simulink model "td1jacobian"  (R2024a)
settings: Solver=FixedStepAuto  StartTime=0.0  StopTime=10.0  FixedStep=0.01  RelTol=1e-3
settings Model: Creator=tr_nguye  LastModifiedBy=tr_nguye

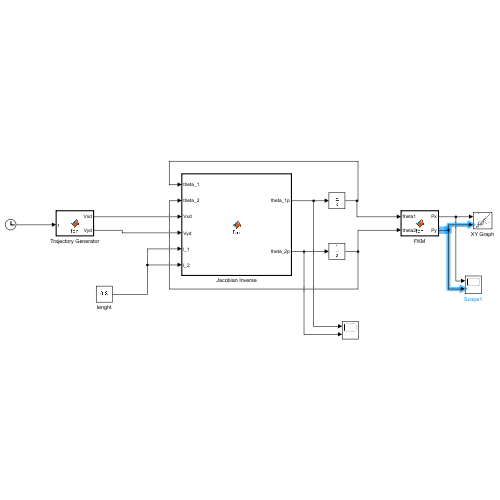
[thumbnail: Simulink's stored preview of the top-level diagram]
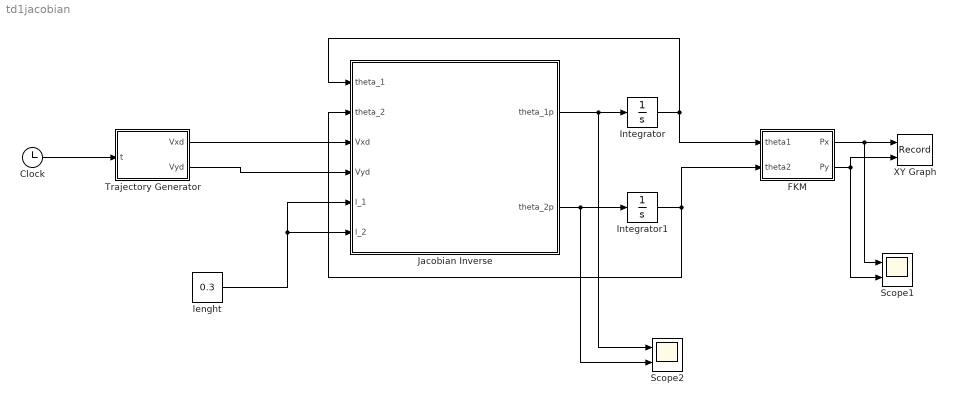
== system td1jacobian ==
  Clock : Clock
      settings: Decimation=1000
  FKM : MATLAB Function  TreatAsAtomicUnit=on
  Integrator : Integrator  InitialCondition=-1.2683
  Integrator1 : Integrator  InitialCondition=0.4759
  Jacobian Inverse : MATLAB Function  TreatAsAtomicUnit=on
  Scope1 : Scope  NumInputPorts=2
  Scope2 : Scope  NumInputPorts=2
  Trajectory Generator : MATLAB Function  TreatAsAtomicUnit=on
  XY Graph : Record  FileSettingsInternal="{\"entries\":[{\"content\":{\"excelSettings\":{\"content\":{},\"type\":\"Streamout.ExcelSettings\"}},\"type\":\"Streamout.FileSettingStorage\",\"uuid\":\"\"}],\"packageUris\":[\"http:\\/\\/schema.mathworks.com\\/mf0\\/streamout_blocks\\/R2020a\"],\"version\":\"1.0\"}"  Layout=[1 1]  SignalsInternal="{\"entries\":[{\"content\":{\"signals\":[{\"content\":{\"blockPath\":[],\"dimensions\":[1],\"domain\":\"\",\"lineColor\":\"#a2142f\",\"plots\":[ 1 ],\"port\":1,\"sid\":[\"\"],\"signalID\":1,\"signalName\":\"FKM:1\"},\"type\":\"RecordBlkView.Signal\",\"uuid\":\"\"},{\"content\":{\"blockPath\":[],\"dimensions\":[1],\"domain\":\"\",\"lineColor\":\"#139fff\",\"plots\":[ 1 ],\"port\":2,\"sid\":[\"\"],\"signalID\":2,\"signalName\":\"FKM:2\"},\"type\":\"RecordBlkView.Signal\",\"uuid\":\"\"}]},\"type\":\"RecordBlkView.InputSignals\",\"uuid\":\"\"}],\"packageUris\":[\"http:\\/\\/schema.mathworks.com\\/mf0\\/streamout_blocks\\/R2020a\"],\"version\":\"1.0\"}"  VisualizationBindings="{\"xyplotplugin\":{\"info\":[{\"series\":[{\"bindingParametersList\":[{\"parameter\":\"X-Axis\",\"signalID\":1,\"signalName\":\"FKM:1\"},{\"parameter\":\"Y-Axis\",\"signalID\":2,\"signalName\":\"FKM:2\"}],\"seriesID\":0}],\"subplotID\":1}]}}"  CompatibilityTag=XY
  lenght : Constant  Value=0.3
  wires:
  Clock/1 -> Trajectory Generator/1(t)
  lenght/1 -> Jacobian Inverse/6(l_2), Jacobian Inverse/5(l_1)
  Jacobian Inverse/1(theta_1p) -> Scope2/1, Integrator/1
  Jacobian Inverse/2(theta_2p) -> Scope2/2, Integrator1/1
  Trajectory Generator/1(Vxd) -> Jacobian Inverse/3(Vxd)
  Trajectory Generator/2(Vyd) -> Jacobian Inverse/4(Vyd)
  Integrator/1 -> FKM/1(theta1), Jacobian Inverse/1(theta_1)
  Integrator1/1 -> FKM/2(theta2), Jacobian Inverse/2(theta_2)
  FKM/1(Px) -> XY Graph/1, Scope1/1
  FKM/2(Py) -> Scope1/2, XY Graph/2

== matlab function td1jacobian/Trajectory Generator ==
  data: t input; Vxd output; Vyd output
function [Vxd, Vyd]= fcn(t)
V = 0.5;
A =  2;
tau = V/A;

x_0 = -0.5;
x_1 = 0.5;

T = abs(x_1 - x_0)/V - tau;

Vxd = 0;
Vyd = 0;
if (t >= 0) && (t <= tau)
    Vyd = A * t;
elseif (t >= tau) && (t <= tau+ T)
    Vyd = V;
elseif (t >= T + tau) && (t <= T + 2*tau)
    Vyd = -A*(t-2*tau-T);
else
    Vyd = 0;
end

== matlab function td1jacobian/Jacobian Inverse ==
  data: theta_1 input; theta_2 input; Vxd input; theta_1p output; theta_2p output; Vyd input; l_1 input; l_2 input
function [theta_1p, theta_2p]= fcn(theta_1, theta_2, Vxd, Vyd, l_1, l_2)
J_nodet = [l_2*cos(theta_1+theta_2) l_2*sin(theta_1+theta_2);
        -l_1*cos(theta_1)-l_2*cos(theta_1+theta_2) -l_1*sin(theta_1)-l_2*sin(theta_1+theta_2)];
det = l_1*l_2*sin(theta_2);

J = (1/det)*J_nodet;


V = [Vxd;Vyd];
theta_p = J * V;

theta_1p = theta_p(1);
theta_2p = theta_p(2);

== matlab function td1jacobian/FKM ==
  data: theta1 input; Px output; Py output; theta2 input
function [Px, Py] = fcn(theta1, theta2)
l_1 = 0.3;
l_2 = 0.3;
Px = l_1*cos(theta1) + l_2*cos(theta1 + theta2);
Py = l_1*sin(theta1) + l_2*sin(theta1 + theta2);
